simulink model "QPSK2"  (Simulink 8.0)
settings: Solver=ode45  StartTime=0.0  StopTime=0.128  RelTol=1e-3
libraries: commrandsrc2 x2, commseqgen2 x1
settings Model: Creator=Dimav  LastModifiedBy=Dimav

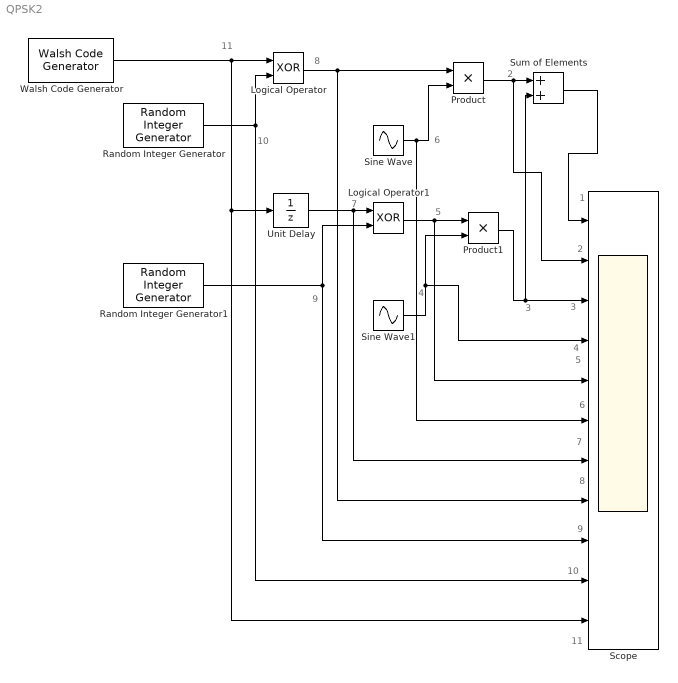
== system QPSK2 ==
  note: 2
  note: 3
  note: 1
  note: 3
  note: 4
  note: 5
  note: 6
  note: 7
  note: 8
  note: 9
  note: 10
  note: 11
  note: 11
  note: 10
  note: 9
  note: 8
  note: 7
  note: 6
  note: 5
  note: 4
  note: 2
  Logical Operator : Logic  Operator=XOR  AllPortsSameDT=off  OutDataTypeStr=boolean
  Logical Operator1 : Logic  Operator=XOR  AllPortsSameDT=off  OutDataTypeStr=boolean
  Product : Product  RndMeth=Zero
  Product1 : Product  RndMeth=Zero
  Random Integer Generator : commrandsrc2/Random Integer Generator  mul=2  seed=12653  Ts=1/1.2288/10^6  frameBased=off  sampPerFrame=1  orient=off  outDataType=double
  Random Integer Generator1 : commrandsrc2/Random Integer Generator  mul=2  seed=21265  Ts=1/1.2288/10^6  frameBased=off  sampPerFrame=1  orient=off  outDataType=double
  Scope : Scope  NumInputPorts=11
      settings: YMin=0~0~0~0.3~0~0.3~-5~-5~-5~-5~-5  YMax=2~1~1~1~1~1~5~5~5~5~5
  Sine Wave : Sin  SampleTime=0
  Sine Wave1 : Sin  SampleTime=0
  Sum of Elements : Sum  Inputs=2
  Unit Delay : UnitDelay  SampleTime=-1
  Walsh Code Generator : commseqgen2/Walsh Code Generator  length=64  index=53  ts=1/1.2288/10^6  frameBased=off  sampPerFrame=1  outDataType=double
  wires:
  Walsh Code Generator/1 -> Unit Delay/1, Scope/11, Logical Operator/1
  Random Integer Generator/1 -> Logical Operator/2, Scope/10
  Unit Delay/1 -> Scope/7, Logical Operator1/1
  Random Integer Generator1/1 -> Logical Operator1/2, Scope/9
  Logical Operator/1 -> Product/1, Scope/8
  Sine Wave/1 -> Product/2, Scope/6
  Logical Operator1/1 -> Scope/5, Product1/1
  Sine Wave1/1 -> Product1/2, Scope/4
  Product1/1 -> Scope/3, Sum of Elements/2
  Product/1 -> Scope/2, Sum of Elements/1
  Sum of Elements/1 -> Scope/1
